simulink model "Step"  (R2025a)
settings: Solver=ode4  StartTime=Tstart  StopTime=Tend  FixedStep=Tsim  RelTol=1e-3
values from neighbouring files (symbols this model uses):
  den = [1, p]    [Motor_Validation.m]
  Ts = 0.005    [Motor_Validation.m]
settings Model: Creator=USER  LastModifiedBy=Ryuminseo
settings OptimizationCC: ReuseModelBlockBuffer=off
settings RTWCC: GPUComputeCapability=3.5

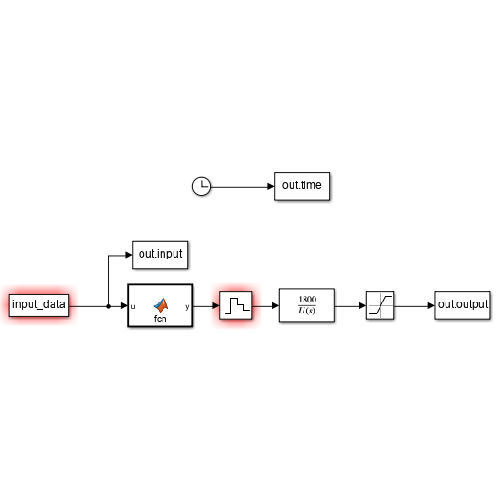
[thumbnail: Simulink's stored preview of the top-level diagram]
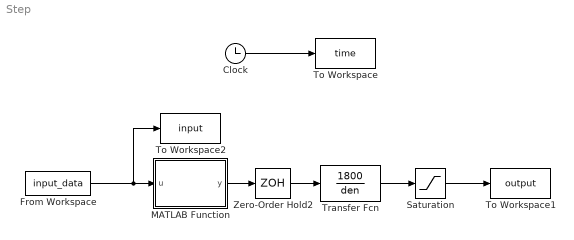
== system Step ==
  Clock : Clock
  From Workspace : FromWorkspace  VariableName=input_data  SampleTime=Ts
  MATLAB Function : MATLAB Function  TreatAsAtomicUnit=on
  Saturation : Saturate  UpperLimit=2.5  LowerLimit=-2.5
  To Workspace : ToWorkspace  VariableName=time  SampleTime=-1
  To Workspace1 : ToWorkspace  VariableName=output  SampleTime=-1
  To Workspace2 : ToWorkspace  VariableName=input  SampleTime=-1
  Transfer Fcn : TransferFcn  Numerator=1800  Denominator=den
  Zero-Order Hold2 : ZeroOrderHold  SampleTime=Ts
  wires:
  From Workspace/1 -> MATLAB Function/1(u), To Workspace2/1
  MATLAB Function/1(y) -> Zero-Order Hold2/1
  Clock/1 -> To Workspace/1
  Saturation/1 -> To Workspace1/1
  Zero-Order Hold2/1 -> Transfer Fcn/1
  Transfer Fcn/1 -> Saturation/1

== matlab function Step/MATLAB Function ==
  data: u input; y output
function y = fcn(u)

    if u >= -0.1 && u <= 0.1
        y = 0;
        
    else
        y = u;
    end
end
